simulink library "NeuroMuscularLibrary2"  (R2019b)
settings: Solver=ode45  StartTime=0.0  StopTime=10.0  RelTol=1e-3  EnableMultiTasking=on
values from neighbouring files (symbols this model uses):
  c = 0.05    [BodyMechParams.m]
  c_jointstop = 0.3 / (pi/180)    (= 17.1887338539)    [BodyMechParams.m]
  deltaLegAngleThr = 8*pi/180    (= 0.13962634016)    [CMGParams.m]
  DeltaThRef = 2e-3    (= 0.002)    [BodyMechParams.m]
  eref = 0.04    [BodyMechParams.m]
  FmaxGLU = 1500    [BodyMechParams.m]
  footBallToAnkleDist = 0.16    [BodyMechParams.m]
  footBallToCenterDist = footLength/2    (= 0.1)    [BodyMechParams.m]
  footBallToHeelDist = footLength    (= 0.2)    [BodyMechParams.m]
  footCenterToCGDist = 0.14 - footBallToCenterDist    (= 0.04)    [BodyMechParams.m]
  footInertia = 0.005    [BodyMechParams.m]
  footLength = 0.2    [BodyMechParams.m]
  footMass = 1.25    [BodyMechParams.m]
  FT_GLU = 47.6    [BodyMechParams.m]
  g = 9.80665    [BodyMechParams.m]
  groundTheta = [atan(diff(groundZ)./diff(groundX)), 0]    [generateGround.m]
  groundZ = groundZ * stepSize/(largestStep+eps)    [generateGround.m]
  hatHipToCenterDistLen = hatLength/2    (= 0.4)    [BodyMechParams.m]
  hatInertia = 3    [BodyMechParams.m]
  hatLeftHipToCenterDistWidth = .15    (= 0.15)    [BodyMechParams.m]
  hatLength = 0.8    [BodyMechParams.m]
  hatMass = 53.5    [BodyMechParams.m]
  hatThickness = 0.2    [BodyMechParams.m]
  hatWidth = 0.4    [BodyMechParams.m]
  K = 5    [BodyMechParams.m]
  k_gn = k_gn/2    (= 39226.6)    [BodyMechParams.m]
  k_gt = k_gt/2    (= 39226.6)    [BodyMechParams.m]
  k_pressure = hatMass * g / DeltaThRef    (= 262327.8875)    [BodyMechParams.m]
  legAngleSpeedMax = 10    [CMGParams.m]
  loptGAS = 0.05    [BodyMechParams.m]
  loptGLU = 0.11    [BodyMechParams.m]
  loptHAB = 0.09    [BodyMechParams.m]
  loptHAD = 0.10    (= 0.1)    [BodyMechParams.m]
  loptHAM = 0.10    (= 0.1)    [BodyMechParams.m]
  loptHFL = 0.11    [BodyMechParams.m]
  loptSOL = 0.04    [BodyMechParams.m]
  loptTA = 0.06    [BodyMechParams.m]
  loptVAS = 0.08    [BodyMechParams.m]
  lslackGAS = 0.40    (= 0.4)    [BodyMechParams.m]
  lslackGLU = 0.13    [BodyMechParams.m]
  lslackHAB = 0.07    [BodyMechParams.m]
  lslackHAD = 0.18    [BodyMechParams.m]
  lslackHAM = 0.31    [BodyMechParams.m]
  lslackHFL = 0.10    (= 0.1)    [BodyMechParams.m]
  lslackSOL = 0.26    [BodyMechParams.m]
  lslackTA = 0.24    [BodyMechParams.m]
  lslackVAS = 0.23    [BodyMechParams.m]
  mu_slide = 0.8    [BodyMechParams.m]
  mu_stick = 0.9    [BodyMechParams.m]
  N = 1.5    [BodyMechParams.m]    (also in cmaes.m = size(x,1); mergeCompareEnergyCosts.m = {S.name})
  phiKneeUpLimit = 5*pi/180    (= 0.0872664625997)    [BodyMechParams.m]
  phimaxGASa = 20*pi/180    (= 0.349065850399)    [BodyMechParams.m]
  phimaxGASk = 40*pi/180    (= 0.698131700798)    [BodyMechParams.m]
  phimaxHAMk = 0*pi/180    (= 0)    [BodyMechParams.m]
  phimaxSOL = 20*pi/180    (= 0.349065850399)    [BodyMechParams.m]
  phimaxTA = -10*pi/180    (= -0.174532925199)    [BodyMechParams.m]
  phimaxVAS = 15*pi/180    (= 0.261799387799)    [BodyMechParams.m]
  phirefGASa = -10*pi/180    (= -0.174532925199)    [BodyMechParams.m]
  phirefGASk = 15*pi/180    (= 0.261799387799)    [BodyMechParams.m]
  phirefGLU = -30*pi/180    (= -0.523598775598)    [BodyMechParams.m]
  phirefHAB = 10*pi/180    (= 0.174532925199)    [BodyMechParams.m]
  phirefHAD = 15*pi/180    (= 0.261799387799)    [BodyMechParams.m]
  phirefHAMh = -25*pi/180    (= -0.436332312999)    [BodyMechParams.m]
  phirefHAMk = 0*pi/180    (= 0)    [BodyMechParams.m]
  phirefHFL = 0*pi/180    (= 0)    [BodyMechParams.m]
  phirefSOL = -10*pi/180    (= -0.174532925199)    [BodyMechParams.m]
  phirefTA = 20*pi/180    (= 0.349065850399)    [BodyMechParams.m]
  phirefVAS = 55*pi/180    (= 0.959931088597)    [BodyMechParams.m]
  rGASa = 0.05    [BodyMechParams.m]
  rGASk = 0.05    [BodyMechParams.m]
  rGLU = 0.10    (= 0.1)    [BodyMechParams.m]
  rHAB = 0.06    [BodyMechParams.m]
  rHAD = 0.03    [BodyMechParams.m]
  rHAMh = 0.08    [BodyMechParams.m]
  rHAMk = 0.05    [BodyMechParams.m]
  rHFL = 0.10    (= 0.1)    [BodyMechParams.m]
  rhoGASa = 0.7    [BodyMechParams.m]
  rhoGASk = 0.7    [BodyMechParams.m]
  rhoGLU = 0.5    [BodyMechParams.m]
  rhoHAB = 0.7    [BodyMechParams.m]
  rhoHAD = 1    [BodyMechParams.m]
  rhoHAMh = 0.7    [BodyMechParams.m]
  rhoHAMk = 0.7    [BodyMechParams.m]
  rhoHFL = 0.5    [BodyMechParams.m]
  rhoSOL = 0.5    [BodyMechParams.m]
  rhoTA = 0.7    [BodyMechParams.m]
  rhoVAS = 0.7    [BodyMechParams.m]
  RkneeExtendGain = 25000    [CMGParams.m]
  RkneeStopGain = 12000    [CMGParams.m]
  RlegAngleFilter = 100    [CMGParams.m]
  rSOL = 0.05    [BodyMechParams.m]
  rTA = 0.04    [BodyMechParams.m]
  rVAS = 0.06    [BodyMechParams.m]
  s = x(1:N-1,:).^2 + x(2:N,:).^2    [cmaes.m]
  shankAnkleToCenterDist = shankLength/2    (= 0.25)    [BodyMechParams.m]
  shankAnkleToKneeDist = shankLength    (= 0.5)    [BodyMechParams.m]
  shankCenterToCGDist = 0.3 - shankAnkleToCenterDist    (= 0.05)    [BodyMechParams.m]
  shankInertia = 0.05    [BodyMechParams.m]
  shankLength = 0.5    [BodyMechParams.m]
  shankMass = 3.5    [BodyMechParams.m]
  tau = 0.01    [BodyMechParams.m]
  thighCenterToCGDist = 0.3 - thighKneeToCenterDist    (= 0.05)    [BodyMechParams.m]
  thighInertia = 0.15    [BodyMechParams.m]
  thighKneeToCenterDist = thighLength/2    (= 0.25)    [BodyMechParams.m]
  thighKneeToHipDist = thighLength    (= 0.5)    [BodyMechParams.m]
  thighLength = 0.5    [BodyMechParams.m]
  thighMass = 8.5    [BodyMechParams.m]
  v_gn_max = v_gz_max    (= 0.03)    [BodyMechParams.m]
  v_gt_max = v_gz_max    (= 0.03)    [BodyMechParams.m]
  v_max_pressure = 0.5    [BodyMechParams.m]
  vLimit = 0.01    [BodyMechParams.m]
  w = 0.56    [BodyMechParams.m]    (also in MuscleEnergyTest.m = 1.039; cmaes.m = ones(size(x,1)))
  w_max_jointstop = 1 * pi/180    (= 0.0174532925199)    [BodyMechParams.m]
  X = contains(N,'compareEnergyCost') .* ~contains(N,'total') .* ~contains(N,'Total')    [mergeCompareEnergyCosts.m]
undefined symbols (not defined in the file or in its folder): abdHATRef, ankleBackDriveGain, ankleCJointstop, ankleDgain, ankleFilterPID, ankleFilterSEA, ankleGearEff, ankleGearRatio, ankleIgain, ankleInitialAngle, ankleInputMass, ankleIntCoulomb, ankleIntDamping, ankleIntStatic, ankleParallelSpringDamping, ankleParallelSpringOffset, ankleParallelSpringStiffness, anklePgain, anklePlantarLimit, ankleSEADamping, ankleSEAStiffness, ankleTendonMass, ankleWMaxJointstop, dryFrictionDamping, dryFrictionStiffness, dryFrictionVelThresh, footMassp, FourBarL1, FourBarL3, GainCHAB, GainCHAD, GainGAS, GainGLU, GainHAM, GainKneeOverExt, GainSOL, GainSOLTA, GainTA, GainVAS, hipDGain, hipDGainAbd, hipPGain, hipPGainAbd, Kglu, kneeAngleOffset, kneeBackDriveGain, kneeCJointstop, kneeDgain, kneeExtCoulomb, kneeExtDamping, kneeExtendGain, kneeExtStatic, kneeFilterPID, kneeFilterSEA, kneeFlexGain, kneeGearEff, kneeGearRatio, kneeHoldGain1, kneeHoldGain2, kneeIgain ... (+62)
libraries: sm_lib x105, nesl_utility x55, simulink x22, dspswit3 x15, $bdroot x12, simulink_extras x2
(part 6 of 6)

== system NeuroMuscularLibrary2/Hill Muscle/CE inverse force-velocity relation ==
  note: CE Inverse Force-Velocity Relationship
  Fv[Fmax] : Inport
  1 : Product  Inputs=/*
  Constant{1,3..4,8} (4 alike) : Constant
  Constant2 : Constant  Value=N
  Constant5 : Constant  Value=N
  Curvature : Gain  Gain=K  SaturateOnIntegerOverflow=on  OutDataTypeStr=Inherit: Same as input  ParamDataTypeStr=Inherit: Same as input
  Curvature1 : Gain  Gain=7.56*K  SaturateOnIntegerOverflow=on  OutDataTypeStr=Inherit: Same as input  ParamDataTypeStr=Inherit: Same as input
  Mux : Mux  Inputs=2
  Mux1 : Mux  Inputs=3
  Mux2 : Mux  Inputs=3
  Slope : Gain  Gain=1e-2  SaturateOnIntegerOverflow=on  OutDataTypeStr=Inherit: Same as input  ParamDataTypeStr=Inherit: Same as input
  Sum1 : Sum  Inputs=|++  SaturateOnIntegerOverflow=on  InputSameDT=on  OutDataTypeStr=Inherit: Same as first input
  Sum2 : Sum  SaturateOnIntegerOverflow=on  InputSameDT=on  OutDataTypeStr=Inherit: Same as first input
  Sum3 : Sum  Inputs=++|  SaturateOnIntegerOverflow=on  InputSameDT=on  OutDataTypeStr=Inherit: Same as first input
  Sum4 : Sum  Inputs=|+-  SaturateOnIntegerOverflow=on  InputSameDT=on  OutDataTypeStr=Inherit: Same as first input
  Sum5 : Sum  Inputs=|-+  SaturateOnIntegerOverflow=on  InputSameDT=on  OutDataTypeStr=Inherit: Same as first input
  Sum6 : Sum  Inputs=-+|  SaturateOnIntegerOverflow=on  InputSameDT=on  OutDataTypeStr=Inherit: Same as first input
  Sum7 : Sum  Inputs=|++  SaturateOnIntegerOverflow=on  InputSameDT=on  OutDataTypeStr=Inherit: Same as first input
  Sum8 : Sum  Inputs=+-|  SaturateOnIntegerOverflow=on  InputSameDT=on  OutDataTypeStr=Inherit: Same as first input
  Sum9 : Sum  SaturateOnIntegerOverflow=on  InputSameDT=on  OutDataTypeStr=Inherit: Same as first input
  concentric branch : Fcn  Expr=u(1) * (u(2)<=1)
  excentric branch : Fcn  Expr=u(2) * (u(1)>1)*(u(1)<=u(3))
  excentric overshoot : Fcn  Expr=u(3) * (u(2)>u(1))
  v_concentric : Product  Inputs=*/
  v_excentric <N : Product  Inputs=*/
  v[vmax] : Outport
  wires:
  Curvature/1 -> Sum3/2
  Constant1/1 -> Sum4/2, Sum3/1
  Sum4/1 -> v_concentric/1
  Sum3/1 -> v_concentric/2
  1/1 -> Sum7/1, Curvature1/1
  Constant4/1 -> Sum7/2, Sum8/1
  Curvature1/1 -> Sum8/2
  Sum8/1 -> v_excentric <N/2
  Sum7/1 -> v_excentric <N/1
  v_concentric/1 -> Mux/1
  Fv[Fmax]/1 -> Sum4/1, Curvature/1, Sum6/2, Mux/2, Mux1/1, Mux2/2
  Sum9/1 -> v[vmax]/1
  Sum2/1 -> Sum9/2
  excentric overshoot/1 -> Sum2/2
  Slope/1 -> Sum1/1
  Constant8/1 -> Sum1/2
  Sum6/1 -> 1/2, Slope/1
  Constant2/1 -> Sum6/1, Sum5/2
  Sum5/1 -> 1/1
  Constant3/1 -> Sum5/1
  Mux/1 -> concentric branch/1
  Mux1/1 -> excentric branch/1
  v_excentric <N/1 -> Mux1/2
  Mux2/1 -> excentric overshoot/1
  concentric branch/1 -> Sum9/1
  excentric branch/1 -> Sum2/1
  Constant5/1 -> Mux1/3, Mux2/1
  Sum1/1 -> Mux2/3

== system NeuroMuscularLibrary2/Hill Muscle/PE force-length relation ==
  note: Parallel Elasticity PE
  lce [lopt] : Inport
  Constant3 : Constant
  Math Function2 : Math  Operator=square  SaturateOnIntegerOverflow=on
  Mux : Mux  Inputs=2
  Sum1 : Sum  Inputs=|+-  SaturateOnIntegerOverflow=on  InputSameDT=on  OutDataTypeStr=Inherit: Same as first input
  force above slack length : Fcn  Expr=u(2) * (u(1)>1)
  reference strain [lopt] : Constant  Value=w
  relative strain : Product  Inputs=*/
  fpe [Fmax] : Outport
  wires:
  Mux/1 -> force above slack length/1
  lce [lopt]/1 -> Mux/1, Sum1/1
  Constant3/1 -> Sum1/2
  Sum1/1 -> relative strain/1
  reference strain [lopt]/1 -> relative strain/2
  relative strain/1 -> Math Function2/1
  Math Function2/1 -> Mux/2
  force above slack length/1 -> fpe [Fmax]/1

== system NeuroMuscularLibrary2/Hill Muscle/SE force-length relation ==
  note: SE Force-Length Relationship
  lse [lslack] : Inport
  Constant1 : Constant
  Math Function : Math  Operator=square  SaturateOnIntegerOverflow=on
  Mux : Mux  Inputs=2
  Sum4 : Sum  Inputs=|+-  SaturateOnIntegerOverflow=on  InputSameDT=on  OutDataTypeStr=Inherit: Same as first input
  force above slack length : Fcn  Expr=u(2)*(u(1)>1)
  reference strain [lslack] : Constant  Value=eref
  relative strain : Product  Inputs=*/
  fse [Fmax] : Outport
  wires:
  Mux/1 -> force above slack length/1
  force above slack length/1 -> fse [Fmax]/1
  Math Function/1 -> Mux/2
  lse [lslack]/1 -> Mux/1, Sum4/1
  relative strain/1 -> Math Function/1
  reference strain [lslack]/1 -> relative strain/2
  Sum4/1 -> relative strain/1
  Constant1/1 -> Sum4/2

== system NeuroMuscularLibrary2/Swing Phase/Filtered Derivative ==
  In1 : Inport
  Filter Coeff : Gain  Gain=legAngleFilter
  Integrator : Integrator
  Sum4 : Sum  Inputs=|+-
  Out1 : Outport
  wires:
  Integrator/1 -> Sum4/2
  Sum4/1 -> Filter Coeff/1
  Filter Coeff/1 -> Integrator/1, Out1/1
  In1/1 -> Sum4/1

== system NeuroMuscularLibrary2/Swing Phase/Knee Flex ==
  LegAngleSpeed : Inport
  Enable : EnablePort  StatesWhenEnabling=reset  ZeroCross=off
  " 4" : Gain  Gain=-kneeFlexGain
  Saturation : Saturate  UpperLimit=0  LowerLimit=-inf  ZeroCross=off
  tau : Outport  OutputWhenDisabled=reset  InitialOutput=0
  wires:
  LegAngleSpeed/1 -> Saturation/1
  " 4"/1 -> tau/1
  Saturation/1 -> " 4"/1

== system NeuroMuscularLibrary2/Swing Phase/Knee Hold ==
  legAngleSpeed : Inport
  legAngle : Inport  Port=2
  legAngleTgt : Inport  Port=3
  kneeSpeed : Inport  Port=4
  Enable : EnablePort  StatesWhenEnabling=reset  ZeroCross=off
  " 5" : Gain  Gain=-kneeHoldGain1
  " 6" : Gain  Gain=-kneeHoldGain2
  Add4 : Sum
  Compare To Zero : simulink/Logic and Bit Operations/Compare To Zero  relop=>=  OutDataTypeStr=boolean  ZeroCross=off
  Compare To Zero1 : simulink/Logic and Bit Operations/Compare To Zero  relop=<  OutDataTypeStr=boolean  ZeroCross=off
  Product1 : Product
  Product2 : Product  Inputs=5
  Relational Operator : RelationalOperator  Operator=<  OutDataTypeStr=boolean  ZeroCross=off  RndMeth=Nearest
  Saturation : Saturate  UpperLimit=inf  LowerLimit=0
  Sum1 : Sum  Inputs=+-|
  Sum3 : Sum  Inputs=+-|
  tau : Outport  OutputWhenDisabled=reset  InitialOutput=0
  wires:
  Product1/1 -> Add4/1
  Saturation/1 -> Add4/2
  Add4/1 -> tau/1
  legAngleTgt/1 -> Sum1/2
  legAngle/1 -> Sum1/1
  legAngleSpeed/1 -> Relational Operator/2, Sum3/1
  Product2/1 -> Saturation/1
  Compare To Zero1/1 -> Product2/4
  Sum3/1 -> Product2/3
  Sum1/1 -> Product2/2
  " 6"/1 -> Product2/1
  kneeSpeed/1 -> Relational Operator/1, Compare To Zero1/1, Sum3/2, Compare To Zero/1, " 5"/1, " 6"/1  "knee speed"
  Compare To Zero/1 -> Product1/2
  " 5"/1 -> Product1/1
  Relational Operator/1 -> Product2/5

== system NeuroMuscularLibrary2/Swing Phase/Knee Stop ==
  note: Knee Extend Torque
  legAngleSpeed : Inport
  legAngle : Inport  Port=2
  legAngleTgt : Inport  Port=3
  Leg Length : Inport  Port=4
  Extend? : Inport  Port=5
  Enable : EnablePort  StatesWhenEnabling=reset  ZeroCross=off
  Add : Sum
  Add5 : Sum  Inputs=-+
  Add6 : Sum  Inputs=+-
  Constant10 : Constant
  Constant11 : Constant  Value=legAngleSpeedMax
  Constant12 : Constant  Value=-kneeExtendGain
  Constant13 : Constant  Value=shankLength + thighLength
  Constant9 : Constant  Value=kneeStopGain
  Divide : Product  Inputs=*/
  Divide1 : Product  Inputs=***
  Product4 : Product  Inputs=5
  Relational Operator1 : RelationalOperator  Operator=<  OutDataTypeStr=boolean  ZeroCross=off  RndMeth=Nearest
  Relational Operator2 : RelationalOperator  Operator=<  OutDataTypeStr=boolean  ZeroCross=off  RndMeth=Nearest
  Sum2 : Sum  Inputs=++|
  Sum5 : Sum  Inputs=|-+
  leg angle Threshold : Constant  Value=deltaLegAngleThr
  tau : Outport  OutputWhenDisabled=reset  InitialOutput=0
  wires:
  Extend?/1 -> Divide1/1
  Leg Length/1 -> Sum5/1
  legAngleSpeed/1 -> Divide/1, Relational Operator2/1
  legAngle/1 -> Add5/1, Relational Operator1/1
  legAngleTgt/1 -> Sum2/1
  Add/1 -> tau/1
  Divide1/1 -> Add/2
  Sum5/1 -> Divide1/3
  Constant13/1 -> Sum5/2
  Constant12/1 -> Divide1/2
  Product4/1 -> Add/1
  Relational Operator2/1 -> Product4/5
  Relational Operator1/1 -> Product4/4
  Divide/1 -> Add6/2
  Constant10/1 -> Add6/1
  Add6/1 -> Product4/2
  Constant11/1 -> Divide/2, Relational Operator2/2
  Constant9/1 -> Product4/3
  Add5/1 -> Product4/1
  Sum2/1 -> Relational Operator1/2, Add5/2
  leg angle Threshold/1 -> Sum2/2

== system NeuroMuscularLibrary2/Swing Phase/Wait 100 ms to enable ==
  In1 : Inport
  Clock : Clock
  Compare To Constant : simulink/Logic and Bit Operations/Compare To Constant  relop=>  const=.1  OutDataTypeStr=boolean  ZeroCross=off
  Product6 : Product
  Out1 : Outport
  wires:
  Product6/1 -> Out1/1
  Clock/1 -> Compare To Constant/1
  Compare To Constant/1 -> Product6/1
  In1/1 -> Product6/2

== system NeuroMuscularLibrary2/Swing Phase 3D/Filtered Derivative ==
  In1 : Inport
  Filter Coeff : Gain  Gain=legAngleFilter
  Integrator : Integrator
  Sum4 : Sum  Inputs=|+-
  Out1 : Outport
  wires:
  In1/1 -> Sum4/1
  Filter Coeff/1 -> Out1/1, Integrator/1
  Sum4/1 -> Filter Coeff/1
  Integrator/1 -> Sum4/2

== system NeuroMuscularLibrary2/Swing Phase 3D/Knee Flex ==
  LegAngleSpeed : Inport
  Enable : EnablePort  StatesWhenEnabling=reset  ZeroCross=off
  " 4" : Gain  Gain=-kneeFlexGain
  Saturation : Saturate  UpperLimit=0  LowerLimit=-inf  ZeroCross=off
  tau : Outport  OutputWhenDisabled=reset  InitialOutput=0
  wires:
  Saturation/1 -> " 4"/1
  " 4"/1 -> tau/1
  LegAngleSpeed/1 -> Saturation/1

== system NeuroMuscularLibrary2/Swing Phase 3D/Knee Hold ==
  legAngleSpeed : Inport
  legAngle : Inport  Port=2
  legAngleTgt : Inport  Port=3
  kneeSpeed : Inport  Port=4
  Enable : EnablePort  StatesWhenEnabling=reset  ZeroCross=off
  " 5" : Gain  Gain=-kneeHoldGain1
  " 6" : Gain  Gain=-kneeHoldGain2
  Add4 : Sum
  Compare To Zero : simulink/Logic and Bit Operations/Compare To Zero  relop=>=  OutDataTypeStr=boolean  ZeroCross=off
  Compare To Zero1 : simulink/Logic and Bit Operations/Compare To Zero  relop=<  OutDataTypeStr=boolean  ZeroCross=off
  Product1 : Product
  Product2 : Product  Inputs=5
  Relational Operator : RelationalOperator  Operator=<  OutDataTypeStr=boolean  ZeroCross=off  RndMeth=Nearest
  Saturation : Saturate  UpperLimit=inf  LowerLimit=0
  Sum1 : Sum  Inputs=+-|
  Sum3 : Sum  Inputs=+-|
  tau : Outport  OutputWhenDisabled=reset  InitialOutput=0
  wires:
  Relational Operator/1 -> Product2/5
  " 5"/1 -> Product1/1
  Compare To Zero/1 -> Product1/2
  kneeSpeed/1 -> " 6"/1, " 5"/1, Compare To Zero/1, Sum3/2, Compare To Zero1/1, Relational Operator/1  "knee speed"
  " 6"/1 -> Product2/1
  Sum1/1 -> Product2/2
  Sum3/1 -> Product2/3
  Compare To Zero1/1 -> Product2/4
  Product2/1 -> Saturation/1
  legAngleSpeed/1 -> Sum3/1, Relational Operator/2
  legAngle/1 -> Sum1/1
  legAngleTgt/1 -> Sum1/2
  Add4/1 -> tau/1
  Saturation/1 -> Add4/2
  Product1/1 -> Add4/1

== system NeuroMuscularLibrary2/Swing Phase 3D/Knee Stop ==
  note: Knee Extend Torque
  legAngleSpeed : Inport
  legAngle : Inport  Port=2
  legAngleTgt : Inport  Port=3
  Leg Length : Inport  Port=4
  Extend? : Inport  Port=5
  Enable : EnablePort  StatesWhenEnabling=reset  ZeroCross=off
  Add : Sum
  Add5 : Sum  Inputs=-+
  Add6 : Sum  Inputs=+-
  Constant10 : Constant
  Constant11 : Constant  Value=legAngleSpeedMax
  Constant12 : Constant  Value=-kneeExtendGain
  Constant13 : Constant  Value=shankLength + thighLength
  Constant9 : Constant  Value=kneeStopGain
  Divide : Product  Inputs=*/
  Divide1 : Product  Inputs=***
  Product4 : Product  Inputs=5
  Relational Operator1 : RelationalOperator  Operator=<  OutDataTypeStr=boolean  ZeroCross=off  RndMeth=Nearest
  Relational Operator2 : RelationalOperator  Operator=<  OutDataTypeStr=boolean  ZeroCross=off  RndMeth=Nearest
  Sum2 : Sum  Inputs=++|
  Sum5 : Sum  Inputs=|-+
  leg angle Threshold : Constant  Value=deltaLegAngleThr
  tau : Outport  OutputWhenDisabled=reset  InitialOutput=0
  wires:
  leg angle Threshold/1 -> Sum2/2
  Sum2/1 -> Add5/2, Relational Operator1/2
  Add5/1 -> Product4/1
  Constant9/1 -> Product4/3
  Constant11/1 -> Relational Operator2/2, Divide/2
  Add6/1 -> Product4/2
  Constant10/1 -> Add6/1
  Divide/1 -> Add6/2
  Relational Operator1/1 -> Product4/4
  Relational Operator2/1 -> Product4/5
  Product4/1 -> Add/1
  Constant12/1 -> Divide1/2
  Constant13/1 -> Sum5/2
  Sum5/1 -> Divide1/3
  Divide1/1 -> Add/2
  Add/1 -> tau/1
  legAngleTgt/1 -> Sum2/1
  legAngle/1 -> Relational Operator1/1, Add5/1
  legAngleSpeed/1 -> Relational Operator2/1, Divide/1
  Leg Length/1 -> Sum5/1
  Extend?/1 -> Divide1/1

== system NeuroMuscularLibrary2/Swing Phase 3D/Wait 100 ms to enable ==
  In1 : Inport
  Clock : Clock
  Compare To Constant : simulink/Logic and Bit Operations/Compare To Constant  relop=>  const=.1  OutDataTypeStr=boolean  ZeroCross=off
  Product6 : Product
  Out1 : Outport
  wires:
  In1/1 -> Product6/2
  Compare To Constant/1 -> Product6/1
  Clock/1 -> Compare To Constant/1
  Product6/1 -> Out1/1

== system NeuroMuscularLibrary2/Full Prosthesis/Ankle  Joint/Ankle Plantarflexion Limit ==
  note: Knee/Hip Joint Limits
  phi [rad] : Inport
  dphi [rad/s] : Inport  Port=2
  Compare To Constant : simulink/Logic and Bit Operations/Compare To Constant  relop=<  const=1.0  OutDataTypeStr=boolean  ZeroCross=off
  Compare To Zero : simulink/Logic and Bit Operations/Compare To Zero  relop=>  OutDataTypeStr=boolean  ZeroCross=off
  Constant : Constant
  Gain : Gain  Gain=-1
  Gain1 : Gain  Gain=ext
  Gain2 : Gain  Gain=-ext
  Gain3 : Gain  Gain=c_jointstop
  Gain4 : Gain  Gain=1/w_max_jointstop
  Gain5 : Gain  Gain=ext
  Product : Product  Inputs=4
  Sum : Sum  Inputs=|+-
  Sum1 : Sum  Inputs=|+-
  overextension angle : Constant  Value=phiUpLimit
  M_stop [Nm] : Outport
  wires:
  Sum/1 -> Gain3/1
  Gain1/1 -> Compare To Zero/1, Gain/1
  Gain3/1 -> Gain1/1
  dphi [rad/s]/1 -> Gain4/1
  overextension angle/1 -> Sum/2
  phi [rad]/1 -> Sum/1
  Gain4/1 -> Gain2/1
  Gain2/1 -> Compare To Constant/1, Sum1/2
  Gain5/1 -> M_stop [Nm]/1
  Constant/1 -> Sum1/1
  Gain/1 -> Product/1
  Sum1/1 -> Product/2
  Compare To Constant/1 -> Product/3
  Compare To Zero/1 -> Product/4
  Product/1 -> Gain5/1

== system NeuroMuscularLibrary2/Full Prosthesis/Ankle Motor/Friction ==
  Velocity : Inport
  Abs : Abs  ZeroCross=off
  Add : Sum  Inputs=+++
  Divide : Product  Inputs=*/*
  Gain : Gain  Gain=sigma0
  Gain1 : Gain  Gain=sigma1
  Gain2 : Gain  Gain=Fv
  Gain3 : Gain  Gain=-1
  Integrator : Integrator  ZeroCross=off
  Subtract : Sum  Inputs=+-
  g(v) : Fcn  Expr=(Fc + (Fs - Fc)*exp(-(u/v_s)^2))/sigma0
  Friction Force : Outport
  wires:
  Gain2/1 -> Add/1
  Gain/1 -> Add/2
  Gain1/1 -> Add/3
  Gain3/1 -> Friction Force/1
  Add/1 -> Gain3/1
  Integrator/1 -> Gain/1, Divide/3  "z"
  g(v)/1 -> Divide/2
  Subtract/1 -> Gain1/1, Integrator/1  "dz/dt"
  Divide/1 -> Subtract/2
  Abs/1 -> Divide/1
  Velocity/1 -> Subtract/1, Abs/1, g(v)/1, Gain2/1

== system NeuroMuscularLibrary2/Full Prosthesis/Ankle Motor/Motor Dynamics ==
  Voltage : Inport
  Speed : Inport  Port=2
  1/Inductance : Gain  Gain=1/motorInductance
  Add : Sum  Inputs=+--
  Integrator : Integrator
  Resistance : Gain  Gain=motorResistance
  Saturation : Saturate  UpperLimit=motorMaxCurrent  LowerLimit=-motorMaxCurrent  ZeroCross=off
  Torsional Constant : Gain  Gain=motorTorsionalConst
  back EMF : Gain  Gain=motorBackEMF
  Torque : Outport
  wires:
  Integrator/1 -> Saturation/1
  Saturation/1 -> Torsional Constant/1, Resistance/1  "Current"
  Resistance/1 -> Add/2
  back EMF/1 -> Add/3
  1/Inductance/1 -> Integrator/1  "di/dt"
  Add/1 -> 1/Inductance/1
  Speed/1 -> back EMF/1
  Torsional Constant/1 -> Torque/1  "Torque"
  Voltage/1 -> Add/1

== system NeuroMuscularLibrary2/Full Prosthesis/Ankle SEA Control/4 bar ratio ==
  Ankle Input Angle : Inport
  Tendon Angle : Inport  Port=2
  Ankle Angle : Inport  Port=3
  Add : Sum  Inputs=--+
  Bias1 : Bias  Bias=-atan(16.3/81)
  Bias3 : Bias  Bias=5*pi/2
  Divide : Product  Inputs=*/
  Gain1 : Gain  Gain=-1
  Gain2 : Gain  Gain=-1
  Gain3 : Gain  Gain=-FourBarL3/FourBarL1
  Gain4 : Gain  Gain=-1
  Trigonometric Function : Trigonometry
  Trigonometric Function1 : Trigonometry
  ratio : Outport
  wires:
  Gain1/1 -> Bias3/1
  Bias1/1 -> Add/3
  Bias3/1 -> Trigonometric Function1/1, Add/2
  Ankle Angle/1 -> Gain4/1
  Gain4/1 -> Bias1/1
  Gain3/1 -> ratio/1  "4 bar ratio"
  Gain2/1 -> Add/1
  Ankle Input Angle/1 -> Gain2/1
  Add/1 -> Trigonometric Function/1
  Tendon Angle/1 -> Gain1/1
  Trigonometric Function/1 -> Divide/1
  Trigonometric Function1/1 -> Divide/2
  Divide/1 -> Gain3/1

== system NeuroMuscularLibrary2/Full Prosthesis/Ankle SEA Control/Feed Forward ==
  Motor Speed : Inport
  Load Acceleration : Inport  Port=2
  Desired Actuator Torque : Inport  Port=3
  1/n : Gain  Gain=1/ankleGearRatio
  Back EMF : Gain  Gain=motorBackEMF
  Filter Coeff : Gain  Gain=ankleFilterSEA
  Integrator : Integrator
  K_b*J_m*n : Gain  Gain=ankleBackDriveGain*motorRotorInertia*ankleGearRatio
  R/K_tau : Gain  Gain=motorResistance/motorTorsionalConst
  Sum : Sum  Inputs=+-|
  Sum1 : Sum  Inputs=|+-
  Sum2 : Sum
  Computed Motor Voltage : Outport
  wires:
  Filter Coeff/1 -> Integrator/1
  Sum1/1 -> Filter Coeff/1
  Integrator/1 -> Sum1/2, K_b*J_m*n/1  "Filtered Accel"
  Load Acceleration/1 -> Sum1/1
  Back EMF/1 -> Sum/1
  Sum2/1 -> R/K_tau/1
  R/K_tau/1 -> Sum/2
  Motor Speed/1 -> Back EMF/1
  Desired Actuator Torque/1 -> 1/n/1
  1/n/1 -> Sum2/2
  K_b*J_m*n/1 -> Sum2/1
  Sum/1 -> Computed Motor Voltage/1

== system NeuroMuscularLibrary2/Full Prosthesis/Knee Joint/Friction ==
  Velocity : Inport
  Abs : Abs  ZeroCross=off
  Add : Sum  Inputs=+++
  Divide : Product  Inputs=*/*
  Gain : Gain  Gain=sigma0
  Gain1 : Gain  Gain=sigma1
  Gain2 : Gain  Gain=Fv
  Gain3 : Gain  Gain=-1
  Integrator : Integrator  ZeroCross=off
  Subtract : Sum  Inputs=+-
  g(v) : Fcn  Expr=(Fc + (Fs - Fc)*exp(-(u/v_s)^2))/sigma0
  Friction Force : Outport
  wires:
  Gain2/1 -> Add/1
  Gain/1 -> Add/2
  Gain1/1 -> Add/3
  Gain3/1 -> Friction Force/1
  Add/1 -> Gain3/1
  Integrator/1 -> Gain/1, Divide/3  "z"
  g(v)/1 -> Divide/2
  Subtract/1 -> Gain1/1, Integrator/1  "dz/dt"
  Divide/1 -> Subtract/2
  Abs/1 -> Divide/1
  Velocity/1 -> Subtract/1, Abs/1, g(v)/1, Gain2/1

== system NeuroMuscularLibrary2/Full Prosthesis/Knee Joint/Knee Plantarflexion Limit ==
  note: Knee/Hip Joint Limits
  phi [rad] : Inport
  dphi [rad/s] : Inport  Port=2
  Compare To Constant : simulink/Logic and Bit Operations/Compare To Constant  relop=<  const=1.0  OutDataTypeStr=boolean  ZeroCross=off
  Compare To Zero : simulink/Logic and Bit Operations/Compare To Zero  relop=>  OutDataTypeStr=boolean  ZeroCross=off
  Constant : Constant
  Gain : Gain  Gain=-1
  Gain1 : Gain  Gain=ext
  Gain2 : Gain  Gain=-ext
  Gain3 : Gain  Gain=c_jointstop
  Gain4 : Gain  Gain=1/w_max_jointstop
  Gain5 : Gain  Gain=ext
  Product : Product  Inputs=4
  Sum : Sum  Inputs=|+-
  Sum1 : Sum  Inputs=|+-
  overextension angle : Constant  Value=phiUpLimit
  M_stop [Nm] : Outport
  wires:
  Product/1 -> Gain5/1
  Compare To Zero/1 -> Product/4
  Compare To Constant/1 -> Product/3
  Sum1/1 -> Product/2
  Gain/1 -> Product/1
  Constant/1 -> Sum1/1
  Gain5/1 -> M_stop [Nm]/1
  Gain2/1 -> Sum1/2, Compare To Constant/1
  Gain4/1 -> Gain2/1
  phi [rad]/1 -> Sum/1
  overextension angle/1 -> Sum/2
  dphi [rad/s]/1 -> Gain4/1
  Gain3/1 -> Gain1/1
  Gain1/1 -> Gain/1, Compare To Zero/1
  Sum/1 -> Gain3/1

== system NeuroMuscularLibrary2/Full Prosthesis/Knee Motor/Friction ==
  Velocity : Inport
  Abs : Abs  ZeroCross=off
  Add : Sum  Inputs=+++
  Divide : Product  Inputs=*/*
  Gain : Gain  Gain=sigma0
  Gain1 : Gain  Gain=sigma1
  Gain2 : Gain  Gain=Fv
  Gain3 : Gain  Gain=-1
  Integrator : Integrator  ZeroCross=off
  Subtract : Sum  Inputs=+-
  g(v) : Fcn  Expr=(Fc + (Fs - Fc)*exp(-(u/v_s)^2))/sigma0
  Friction Force : Outport
  wires:
  Gain2/1 -> Add/1
  Gain/1 -> Add/2
  Gain1/1 -> Add/3
  Gain3/1 -> Friction Force/1
  Add/1 -> Gain3/1
  Integrator/1 -> Gain/1, Divide/3  "z"
  g(v)/1 -> Divide/2
  Subtract/1 -> Gain1/1, Integrator/1  "dz/dt"
  Divide/1 -> Subtract/2
  Abs/1 -> Divide/1
  Velocity/1 -> Subtract/1, Abs/1, g(v)/1, Gain2/1

== system NeuroMuscularLibrary2/Full Prosthesis/Knee Motor/Motor Dynamics ==
  Voltage : Inport
  Speed : Inport  Port=2
  1/Inductance : Gain  Gain=1/motorInductance
  Add : Sum  Inputs=+--
  Integrator : Integrator
  Resistance : Gain  Gain=motorResistance
  Saturation : Saturate  UpperLimit=motorMaxCurrent  LowerLimit=-motorMaxCurrent  ZeroCross=off
  Torsional Constant : Gain  Gain=motorTorsionalConst
  back EMF : Gain  Gain=motorBackEMF
  Torque : Outport
  wires:
  Integrator/1 -> Saturation/1
  Saturation/1 -> Torsional Constant/1, Resistance/1  "Current"
  Resistance/1 -> Add/2
  back EMF/1 -> Add/3
  1/Inductance/1 -> Integrator/1  "di/dt"
  Add/1 -> 1/Inductance/1
  Speed/1 -> back EMF/1
  Torsional Constant/1 -> Torque/1  "Torque"
  Voltage/1 -> Add/1

== system NeuroMuscularLibrary2/Full Prosthesis/Knee SEA Control/Feed Forward ==
  Motor Speed : Inport
  Load Acceleration : Inport  Port=2
  Desired Torque : Inport  Port=3
  1/n : Gain  Gain=1/kneeGearRatio
  Back EMF : Gain  Gain=motorBackEMF
  Filter Coeff : Gain  Gain=kneeFilterSEA
  Integrator : Integrator
  K_b*J_m*n : Gain  Gain=kneeBackDriveGain*motorRotorInertia*kneeGearRatio
  R/K_tau : Gain  Gain=motorResistance/motorTorsionalConst
  Sum : Sum  Inputs=+-|
  Sum1 : Sum  Inputs=|+-
  Sum2 : Sum
  Computed Motor Voltage : Outport
  wires:
  Filter Coeff/1 -> Integrator/1
  Sum1/1 -> Filter Coeff/1
  Integrator/1 -> Sum1/2, K_b*J_m*n/1  "Filtered Accel"
  Load Acceleration/1 -> Sum1/1
  Back EMF/1 -> Sum/1
  Sum2/1 -> R/K_tau/1
  R/K_tau/1 -> Sum/2
  Motor Speed/1 -> Back EMF/1
  Desired Torque/1 -> 1/n/1
  1/n/1 -> Sum2/2
  K_b*J_m*n/1 -> Sum2/1
  Sum/1 -> Computed Motor Voltage/1

== system NeuroMuscularLibrary2/Ground Contact Model/2D Contact/Friction Switch ==
  note: Static/Kinetic Friction Switch
  Slide! : Inport
  Stick! : Inport  Port=2
  Memory : Memory
  S-R Flip-Flop : simulink_extras/Flip Flops/S-R Flip-Flop  initial_condition=0
  Terminator : Terminator
  Stiction : Outport
  wires:
  Memory/1 -> Stiction/1
  Slide!/1 -> S-R Flip-Flop/2
  Stick!/1 -> S-R Flip-Flop/1
  S-R Flip-Flop/2 -> Terminator/1
  S-R Flip-Flop/1 -> Memory/1

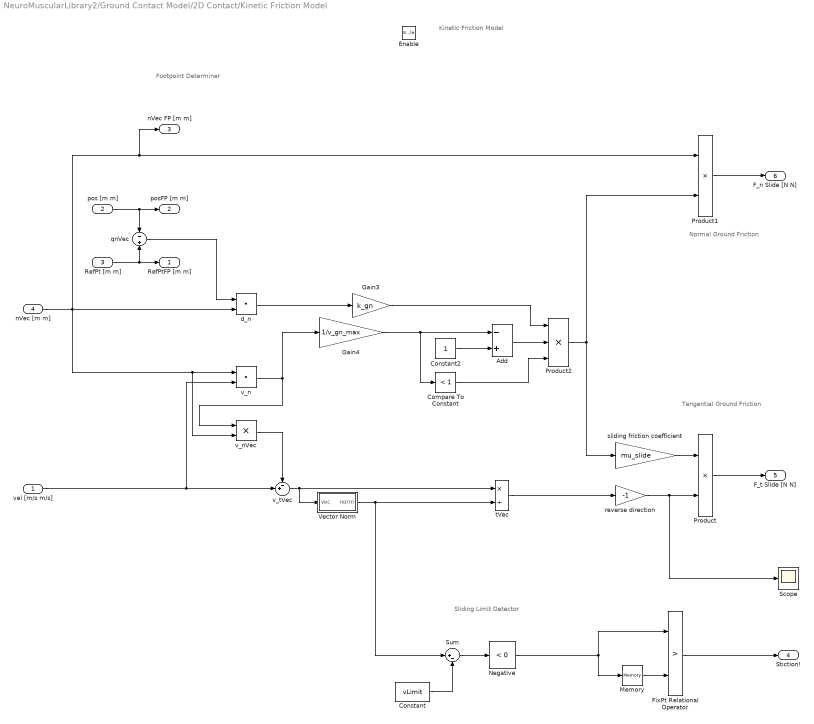
== system NeuroMuscularLibrary2/Ground Contact Model/2D Contact/Kinetic Friction Model ==
  note: Tangential Ground Friction
  note: Normal Ground Friction
  note: Sliding Limit Detector
  note: Footpoint Determiner
  note: Kinetic Friction Model
  vel [m/s m/s] : Inport
  pos [m m] : Inport  Port=2
  RefPt [m m] : Inport  Port=3
  nVec [m m] : Inport  Port=4
  Enable : EnablePort  StatesWhenEnabling=reset  ZeroCross=off
  Add : Sum  Inputs=-+
  Compare To Constant : simulink/Logic and Bit Operations/Compare To Constant  relop=<  const=1  OutDataTypeStr=boolean
  Constant : Constant  Value=vLimit
  Constant2 : Constant
  FixPt Relational Operator : RelationalOperator  Operator=>  OutDataTypeStr=boolean  ZeroCross=off  RndMeth=Nearest
  Gain3 : Gain  Gain=k_gn
  Gain4 : Gain  Gain=1/v_gn_max
  Memory : Memory
  Negative : simulink/Logic and Bit Operations/Compare To Zero  relop=<  OutDataTypeStr=boolean
  Product : Product  RndMeth=Zero
  Product1 : Product  RndMeth=Zero
  Product2 : Product  Inputs=3
  Scope : Scope
  Sum : Sum  Inputs=|+-
  Vector Norm : Subsystem
  d_n : DotProduct  InputSameDT=on  OutDataTypeStr=Inherit: Inherit via internal rule
  qnVec : Sum  Inputs=-+
  reverse direction : Gain  Gain=-1
  sliding friction coefficient : Gain  Gain=mu_slide
  tVec : Product  Inputs=*/  RndMeth=Zero
  v_n : DotProduct  InputSameDT=on  OutDataTypeStr=Inherit: Inherit via internal rule
  v_nVec : Product  RndMeth=Zero
  v_tVec : Sum  Inputs=-+|
  RefPtFP [m m] : Outport  InitialOutput=[0 0]
      settings: AttributesFormatString=initial = '%<InitialOutput>'\nwhen disabled = '%<OutputWhenDisabled>'
  posFP [m m] : Outport  Port=2  InitialOutput=[0 0]
      settings: AttributesFormatString=initial = '%<InitialOutput>'\nwhen disabled = '%<OutputWhenDisabled>'
  nVec FP [m m] : Outport  Port=3  InitialOutput=0
      settings: AttributesFormatString=initial = '%<InitialOutput>'\nwhen disabled = '%<OutputWhenDisabled>'
  Stiction! : Outport  Port=4  OutputWhenDisabled=reset  InitialOutput=0
      settings: AttributesFormatString=initial = '%<InitialOutput>'\nwhen disabled = '%<OutputWhenDisabled>'
  F_t Slide [N N] : Outport  Port=5  OutputWhenDisabled=reset  InitialOutput=[0 0]
      settings: AttributesFormatString=initial = '%<InitialOutput>'\nwhen disabled = '%<OutputWhenDisabled>'
  F_n Slide [N N] : Outport  Port=6  OutputWhenDisabled=reset  InitialOutput=[0 0]
      settings: AttributesFormatString=initial = '%<InitialOutput>'\nwhen disabled = '%<OutputWhenDisabled>'
  wires:
  RefPt [m m]/1 -> RefPtFP [m m]/1, qnVec/2
  qnVec/1 -> d_n/1
  pos [m m]/1 -> qnVec/1, posFP [m m]/1
  tVec/1 -> reverse direction/1
  Product1/1 -> F_n Slide [N N]/1
  reverse direction/1 -> Scope/1, Product/2
  sliding friction coefficient/1 -> Product/1
  v_nVec/1 -> v_tVec/1
  v_n/1 -> v_nVec/1, Gain4/1
  vel [m/s m/s]/1 -> v_tVec/2, v_n/2
  d_n/1 -> Gain3/1
  nVec [m m]/1 -> nVec FP [m m]/1, Product1/1, d_n/2, v_nVec/2, v_n/1
  Constant/1 -> Sum/2
  Sum/1 -> Negative/1
  Vector Norm/1(norm) -> tVec/2, Sum/1
  Product/1 -> F_t Slide [N N]/1
  Product2/1 -> Product1/2, sliding friction coefficient/1
  Gain3/1 -> Product2/1
  Gain4/1 -> Compare To Constant/1, Add/1
  Constant2/1 -> Add/2
  Compare To Constant/1 -> Product2/3
  Add/1 -> Product2/2
  v_tVec/1 -> Vector Norm/1(vec), tVec/1
  FixPt Relational Operator/1 -> Stiction!/1
  Memory/1 -> FixPt Relational Operator/2
  Negative/1 -> FixPt Relational Operator/1, Memory/1

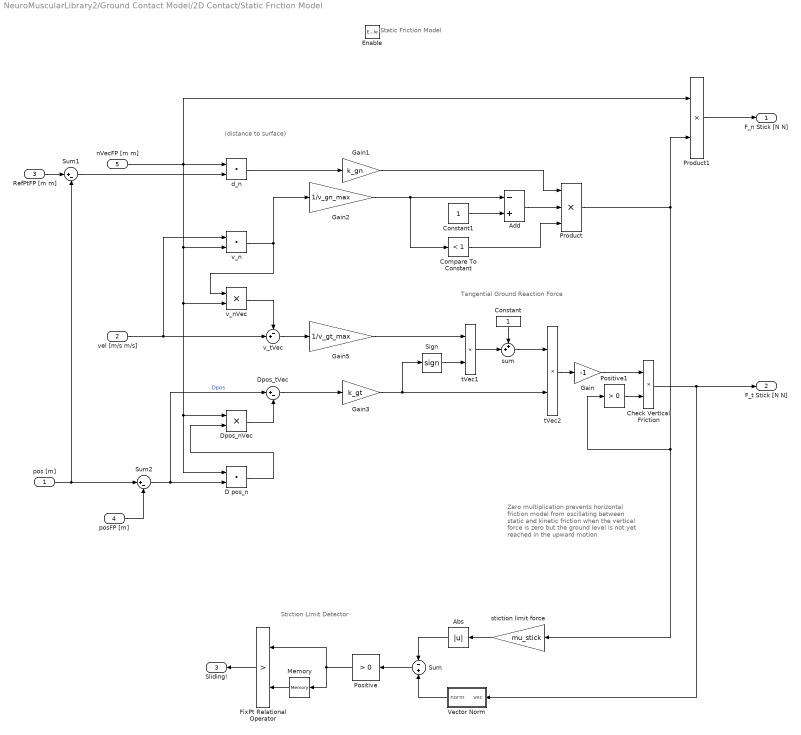
== system NeuroMuscularLibrary2/Ground Contact Model/2D Contact/Static Friction Model ==
  note: Tangential Ground Reaction Force
  note: (distance to
      | surface)
  note: Zero multiplication prevents
      | horizontal friction model from
      | oscillating between static and kinetic
      | friction when the vertical force is zero but
      | the ground level is not yet reached
      | in the upward motion
  note: Static Friction Model
  note: Stiction Limit Detector
  pos [m] : Inport
  vel [m/s m/s] : Inport  Port=2
  RefPtFP [m m] : Inport  Port=3
  posFP [m] : Inport  Port=4
  nVecFP [m m] : Inport  Port=5
  Enable : EnablePort  StatesWhenEnabling=reset  ZeroCross=off
  Abs : Abs
  Add : Sum  Inputs=-+
  Check Vertical Friction : Product  RndMeth=Zero
  Compare To Constant : simulink/Logic and Bit Operations/Compare To Constant  relop=<  const=1  OutDataTypeStr=boolean  ZeroCross=off
  Constant : Constant
  Constant1 : Constant
  D pos_n : DotProduct  InputSameDT=on  OutDataTypeStr=Inherit: Inherit via internal rule
  Dpos_nVec : Product  RndMeth=Zero
  Dpos_tVec : Sum  Inputs=|+-
  FixPt Relational Operator : RelationalOperator  Operator=>  OutDataTypeStr=boolean  ZeroCross=off  RndMeth=Nearest
  Gain : Gain  Gain=-1
  Gain1 : Gain  Gain=k_gn
  Gain2 : Gain  Gain=1/v_gn_max
  Gain3 : Gain  Gain=k_gt
  Gain5 : Gain  Gain=1/v_gt_max
  Memory : Memory
  Positive : simulink/Logic and Bit Operations/Compare To Zero  relop=>  OutDataTypeStr=boolean
  Positive1 : simulink/Logic and Bit Operations/Compare To Zero  relop=>  OutDataTypeStr=boolean
  Product : Product  Inputs=3
  Product1 : Product  RndMeth=Zero
  Sign : Signum  ZeroCross=off
  Sum : Sum  Inputs=-+
  Sum1 : Sum  Inputs=|+-
  Sum2 : Sum  Inputs=|+-
  Vector Norm : Subsystem
  d_n : DotProduct  InputSameDT=on  OutDataTypeStr=Inherit: Inherit via internal rule
  stiction limit force : Gain  Gain=mu_stick
  sum : Sum  Inputs=++|
  tVec1 : Product  Inputs=**  RndMeth=Zero
  tVec2 : Product  Inputs=**  RndMeth=Zero
  v_n : DotProduct  InputSameDT=on  OutDataTypeStr=Inherit: Inherit via internal rule
  v_nVec : Product  RndMeth=Zero
  v_tVec : Sum  Inputs=-+|
  F_n Stick [N N] : Outport  OutputWhenDisabled=reset  InitialOutput=[0 0]
      settings: AttributesFormatString=initial = '%<InitialOutput>'\nwhen disabled = '%<OutputWhenDisabled>'
  F_t Stick [N N] : Outport  Port=2  OutputWhenDisabled=reset  InitialOutput=[0 0]
      settings: AttributesFormatString=when disabled: %<OutputWhenDisabled>\ninitial: %<InitialOutput>
  Sliding! : Outport  Port=3  OutputWhenDisabled=reset  InitialOutput=0
      settings: AttributesFormatString=when disabled: %<OutputWhenDisabled>\ninitial: %<InitialOutput>
  wires:
  Gain5/1 -> tVec1/1
  Sum1/1 -> d_n/2
  RefPtFP [m m]/1 -> Sum1/1
  Vector Norm/1(norm) -> Sum/2
  Gain/1 -> Check Vertical Friction/1
  tVec2/1 -> Gain/1
  sum/1 -> tVec2/1
  Constant/1 -> sum/1
  tVec1/1 -> sum/2
  Sign/1 -> tVec1/2
  Gain3/1 -> tVec2/2, Sign/1
  Dpos_tVec/1 -> Gain3/1
  Dpos_nVec/1 -> Dpos_tVec/2
  D pos_n/1 -> Dpos_nVec/2
  Sum2/1 -> Dpos_tVec/1, D pos_n/2  "Dpos"
  posFP [m]/1 -> Sum2/2
  pos [m]/1 -> Sum1/2, Sum2/1
  Product1/1 -> F_n Stick [N N]/1
  v_tVec/1 -> Gain5/1
  v_nVec/1 -> v_tVec/1
  v_n/1 -> Gain2/1, v_nVec/1
  vel [m/s m/s]/1 -> v_n/1, v_tVec/2
  d_n/1 -> Gain1/1
  nVecFP [m m]/1 -> Product1/1, v_nVec/2, Dpos_nVec/1, D pos_n/1, v_n/2, d_n/1
  Gain1/1 -> Product/1
  Product/1 -> Positive1/1, stiction limit force/1, Product1/2
  Check Vertical Friction/1 -> Vector Norm/1(vec), F_t Stick [N N]/1
  Positive1/1 -> Check Vertical Friction/2
  stiction limit force/1 -> Abs/1
  Abs/1 -> Sum/1
  Sum/1 -> Positive/1
  Gain2/1 -> Compare To Constant/1, Add/1
  Constant1/1 -> Add/2
  Compare To Constant/1 -> Product/3
  Add/1 -> Product/2
  Memory/1 -> FixPt Relational Operator/2
  Positive/1 -> Memory/1, FixPt Relational Operator/1
  FixPt Relational Operator/1 -> Sliding!/1

== system NeuroMuscularLibrary2/Ground Contact Model/2D Contact/Kinetic Friction Model/Vector Norm ==
  vec : Inport
  Constant : Constant  Value=1/2
  Math Function : Math  Operator=pow  SaturateOnIntegerOverflow=on
  Squares : Math  Operator=square  OutputSignalType=real  SaturateOnIntegerOverflow=on
  Sum of Elements : Sum  Inputs=+
  norm : Outport
  wires:
  vec/1 -> Squares/1
  Math Function/1 -> norm/1
  Sum of Elements/1 -> Math Function/1
  Squares/1 -> Sum of Elements/1
  Constant/1 -> Math Function/2

== system NeuroMuscularLibrary2/Ground Contact Model/2D Contact/Static Friction Model/Vector Norm ==
  vec : Inport
  Constant : Constant  Value=1/2
  Math Function : Math  Operator=pow  SaturateOnIntegerOverflow=on
  Squares : Math  Operator=square  OutputSignalType=real  SaturateOnIntegerOverflow=on
  Sum of Elements : Sum  Inputs=+
  norm : Outport
  wires:
  vec/1 -> Squares/1
  Math Function/1 -> norm/1
  Sum of Elements/1 -> Math Function/1
  Squares/1 -> Sum of Elements/1
  Constant/1 -> Math Function/2

== stateflow chart NeuroMuscularLibrary2/Swing Phase/Chart ==
  settings: updateMethod=CONTINUOUS
  state KneeFlexion
    entry: flex = 1;
    exit: flex = 0;
  state KneeHoldStopAndExtend
    entry: hold = 1;
    exit: hold = 0;
    state KneeStopAndExtend
      entry: stop = 1;
      exit: stop = 0;
      state Extend
        entry: extend = 1;
        exit: extend = 0;
      state KneeStopOnly
      KneeStopOnly -> Extend : [legAngleSpeed >= 0]
      (default) -> KneeStopOnly
    state KneeHoldOnly
    KneeHoldOnly -> KneeStopAndExtend : [(legAngle < (legAngleTgt + ...
        | deltaLegAngleThr)) || Stance]
    (default) -> KneeHoldOnly
  KneeHoldStopAndExtend -> KneeFlexion : [Stance]
  KneeFlexion -> KneeHoldStopAndExtend : [(legLength < legLengthClr) && contraStance && ~Stance]
  (default) -> KneeHoldStopAndExtend
  data: Stance input; contraStance input; deltaLegAngleThr parameter; legAngle input; legAngleSpeed input; legAngleTgt input; legLength input; legLengthClr parameter; flex output double; hold output double; stop output double; extend output double

== stateflow chart NeuroMuscularLibrary2/Prosthetic Swing Phase/Chart ==
  settings: updateMethod=CONTINUOUS
  state KneeFlexion
    entry: flex = 1;
    exit: flex = 0;
  state KneeHoldStopAndExtend
    entry: hold = 1;
    exit: hold = 0;
    state KneeStopAndExtend
      entry: stop = 1;
      exit: stop = 0;
      state Extend
        entry: extend = 1;
        exit: extend = 0;
      state KneeStopOnly
      KneeStopOnly -> Extend : [legAngleSpeed >= 0]
      (default) -> KneeStopOnly
    state KneeHoldOnly
    KneeHoldOnly -> KneeStopAndExtend : [(legAngle < (legAngleTgt + ...
        | deltaLegAngleThr)) || Stance]
    (default) -> KneeHoldOnly
  KneeHoldStopAndExtend -> KneeFlexion : [Stance]
  KneeFlexion -> KneeHoldStopAndExtend : [(legLength < legLengthClr) && contraStance && ~Stance]
  (default) -> KneeHoldStopAndExtend
  data: Stance input; contraStance input; deltaLegAngleThr parameter; legAngle input; legAngleSpeed input; legAngleTgt input; legLength input; legLengthClr parameter; flex output double; hold output double; stop output double; extend output double

== stateflow chart NeuroMuscularLibrary2/Swing Phase 3D/Chart ==
  settings: updateMethod=CONTINUOUS
  state KneeFlexion
    entry: flex = 1;
    exit: flex = 0;
  state KneeHoldStopAndExtend
    entry: hold = 1;
    exit: hold = 0;
    state KneeStopAndExtend
      entry: stop = 1;
      exit: stop = 0;
      state Extend
        entry: extend = 1;
        exit: extend = 0;
      state KneeStopOnly
      KneeStopOnly -> Extend : [legAngleSpeed >= 0]
      (default) -> KneeStopOnly
    state KneeHoldOnly
    KneeHoldOnly -> KneeStopAndExtend : [(legAngle < (legAngleTgt + ...
        | deltaLegAngleThr)) || Stance]
    (default) -> KneeHoldOnly
  KneeHoldStopAndExtend -> KneeFlexion : [Stance]
  KneeFlexion -> KneeHoldStopAndExtend : [(legLength < legLengthClr) && contraStance && ~Stance]
  (default) -> KneeHoldStopAndExtend
  data: Stance input; contraStance input; deltaLegAngleThr parameter; legAngle input; legAngleSpeed input; legAngleTgt input; legLength input; legLengthClr parameter; flex output double; hold output double; stop output double; extend output double
